simulink library "Tetris_Lib"  (R2023a)
settings: Solver=ode45  StartTime=0.0  StopTime=10.0  RelTol=1e-3  EnableMultiTasking=on
libraries: simulink_extras x33, $bdroot x16, Bit_Multiplexers_Lib x9, Decoders_Lib x4
(part 2 of 2)

== system Tetris_Lib/Trash_Bin/Shape_Bitmaps/L1-shape (180deg) ==
  note: X
      |
      | Y
      |
      | 0
      | 1
      | 2
      | 3
      |
      | 0
      |
      | 1
      |
      | 2
      |
      | 3
  x3(1b) : Inport
  x2(1b) : Inport  Port=2
  x1(1b) : Inport  Port=3
  x0(1b) : Inport  Port=4
  y3(1b) : Inport  Port=5
  y2(1b) : Inport  Port=6
  y1(1b) : Inport  Port=7
  y0(1b) : Inport  Port=8
  And{,1..3,5..16} (16 alike) : Logic  Inputs=3  IconShape=distinctive  AllPortsSameDT=off  OutDataTypeStr=boolean
  And4 : Logic  Operator=OR  Inputs=16  IconShape=distinctive  AllPortsSameDT=off  OutDataTypeStr=boolean
  None{1..4,8..9,11..16} (12 alike) : Constant  Value=0  OutDataTypeStr=boolean
  None{5..7,10} (4 alike) : Constant  OutDataTypeStr=boolean
  Out(1b) : Outport
  wires:
  y0(1b)/1 -> And/3, And1/3, And6/3, And5/3
  y1(1b)/1 -> And2/3, And3/3, And8/3, And7/3
  x0(1b)/1 -> And/2, And2/2, And11/2, And9/2
  x1(1b)/1 -> And1/2, And3/2, And12/2, And10/2
  And4/1 -> Out(1b)/1
  x2(1b)/1 -> And5/2, And7/2, And15/2, And13/2
  x3(1b)/1 -> And6/2, And8/2, And16/2, And14/2
  y2(1b)/1 -> And9/3, And10/3, And14/3, And13/3
  y3(1b)/1 -> And11/3, And12/3, And16/3, And15/3
  And6/1 -> And4/1
  And5/1 -> And4/2
  And1/1 -> And4/3
  And/1 -> And4/4
  And8/1 -> And4/5
  And7/1 -> And4/6
  And3/1 -> And4/7
  And2/1 -> And4/8
  And14/1 -> And4/9
  And13/1 -> And4/10
  And10/1 -> And4/11
  And9/1 -> And4/12
  And16/1 -> And4/13
  And15/1 -> And4/14
  And12/1 -> And4/15
  And11/1 -> And4/16
  None10/1 -> And/1
  None1/1 -> And2/1
  None2/1 -> And9/1
  None3/1 -> And11/1
  None4/1 -> And12/1
  None5/1 -> And10/1
  None6/1 -> And3/1
  None7/1 -> And1/1
  None8/1 -> And5/1
  None9/1 -> And7/1
  None11/1 -> And13/1
  None12/1 -> And15/1
  None13/1 -> And6/1
  None14/1 -> And8/1
  None15/1 -> And14/1
  None16/1 -> And16/1

== system Tetris_Lib/Trash_Bin/Shape_Bitmaps/L1-shape (270deg) ==
  note: X
      |
      | Y
      |
      | 0
      | 1
      | 2
      | 3
      |
      | 0
      |
      | 1
      |
      | 2
      |
      | 3
  x3(1b) : Inport
  x2(1b) : Inport  Port=2
  x1(1b) : Inport  Port=3
  x0(1b) : Inport  Port=4
  y3(1b) : Inport  Port=5
  y2(1b) : Inport  Port=6
  y1(1b) : Inport  Port=7
  y0(1b) : Inport  Port=8
  And{,1..3,5..16} (16 alike) : Logic  Inputs=3  IconShape=distinctive  AllPortsSameDT=off  OutDataTypeStr=boolean
  And4 : Logic  Operator=OR  Inputs=16  IconShape=distinctive  AllPortsSameDT=off  OutDataTypeStr=boolean
  None{1,6,8..9} (4 alike) : Constant  OutDataTypeStr=boolean
  None{2..5,7,10..16} (12 alike) : Constant  Value=0  OutDataTypeStr=boolean
  Out(1b) : Outport
  wires:
  y0(1b)/1 -> And/3, And1/3, And6/3, And5/3
  y1(1b)/1 -> And2/3, And3/3, And8/3, And7/3
  x0(1b)/1 -> And/2, And2/2, And11/2, And9/2
  x1(1b)/1 -> And1/2, And3/2, And12/2, And10/2
  And4/1 -> Out(1b)/1
  x2(1b)/1 -> And5/2, And7/2, And15/2, And13/2
  x3(1b)/1 -> And6/2, And8/2, And16/2, And14/2
  y2(1b)/1 -> And9/3, And10/3, And14/3, And13/3
  y3(1b)/1 -> And11/3, And12/3, And16/3, And15/3
  And6/1 -> And4/1
  And5/1 -> And4/2
  And1/1 -> And4/3
  And/1 -> And4/4
  And8/1 -> And4/5
  And7/1 -> And4/6
  And3/1 -> And4/7
  And2/1 -> And4/8
  And14/1 -> And4/9
  And13/1 -> And4/10
  And10/1 -> And4/11
  And9/1 -> And4/12
  And16/1 -> And4/13
  And15/1 -> And4/14
  And12/1 -> And4/15
  And11/1 -> And4/16
  None10/1 -> And/1
  None1/1 -> And2/1
  None2/1 -> And9/1
  None3/1 -> And11/1
  None4/1 -> And12/1
  None5/1 -> And10/1
  None6/1 -> And3/1
  None7/1 -> And1/1
  None8/1 -> And5/1
  None9/1 -> And7/1
  None11/1 -> And13/1
  None12/1 -> And15/1
  None13/1 -> And6/1
  None14/1 -> And8/1
  None15/1 -> And14/1
  None16/1 -> And16/1

== system Tetris_Lib/Trash_Bin/Shape_Bitmaps/L1-shape (90deg) ==
  note: X
      |
      | Y
      |
      | 0
      | 1
      | 2
      | 3
      |
      | 0
      |
      | 1
      |
      | 2
      |
      | 3
  x3(1b) : Inport
  x2(1b) : Inport  Port=2
  x1(1b) : Inport  Port=3
  x0(1b) : Inport  Port=4
  y3(1b) : Inport  Port=5
  y2(1b) : Inport  Port=6
  y1(1b) : Inport  Port=7
  y0(1b) : Inport  Port=8
  And{,1..3,5..16} (16 alike) : Logic  Inputs=3  IconShape=distinctive  AllPortsSameDT=off  OutDataTypeStr=boolean
  And4 : Logic  Operator=OR  Inputs=16  IconShape=distinctive  AllPortsSameDT=off  OutDataTypeStr=boolean
  None{1,7..8,10} (4 alike) : Constant  OutDataTypeStr=boolean
  None{2..6,9,11..16} (12 alike) : Constant  Value=0  OutDataTypeStr=boolean
  Out(1b) : Outport
  wires:
  y0(1b)/1 -> And/3, And1/3, And6/3, And5/3
  y1(1b)/1 -> And2/3, And3/3, And8/3, And7/3
  x0(1b)/1 -> And/2, And2/2, And11/2, And9/2
  x1(1b)/1 -> And1/2, And3/2, And12/2, And10/2
  And4/1 -> Out(1b)/1
  x2(1b)/1 -> And5/2, And7/2, And15/2, And13/2
  x3(1b)/1 -> And6/2, And8/2, And16/2, And14/2
  y2(1b)/1 -> And9/3, And10/3, And14/3, And13/3
  y3(1b)/1 -> And11/3, And12/3, And16/3, And15/3
  And6/1 -> And4/1
  And5/1 -> And4/2
  And1/1 -> And4/3
  And/1 -> And4/4
  And8/1 -> And4/5
  And7/1 -> And4/6
  And3/1 -> And4/7
  And2/1 -> And4/8
  And14/1 -> And4/9
  And13/1 -> And4/10
  And10/1 -> And4/11
  And9/1 -> And4/12
  And16/1 -> And4/13
  And15/1 -> And4/14
  And12/1 -> And4/15
  And11/1 -> And4/16
  None10/1 -> And/1
  None1/1 -> And2/1
  None2/1 -> And9/1
  None3/1 -> And11/1
  None4/1 -> And12/1
  None5/1 -> And10/1
  None6/1 -> And3/1
  None7/1 -> And1/1
  None8/1 -> And5/1
  None9/1 -> And7/1
  None11/1 -> And13/1
  None12/1 -> And15/1
  None13/1 -> And6/1
  None14/1 -> And8/1
  None15/1 -> And14/1
  None16/1 -> And16/1

== system Tetris_Lib/Trash_Bin/Shape_Bitmaps/L2-shape (0deg) ==
  note: X
      |
      | Y
      |
      | 0
      | 1
      | 2
      | 3
      |
      | 0
      |
      | 1
      |
      | 2
      |
      | 3
  x3(1b) : Inport
  x2(1b) : Inport  Port=2
  x1(1b) : Inport  Port=3
  x0(1b) : Inport  Port=4
  y3(1b) : Inport  Port=5
  y2(1b) : Inport  Port=6
  y1(1b) : Inport  Port=7
  y0(1b) : Inport  Port=8
  And{,1..3,5..16} (16 alike) : Logic  Inputs=3  IconShape=distinctive  AllPortsSameDT=off  OutDataTypeStr=boolean
  And4 : Logic  Operator=OR  Inputs=16  IconShape=distinctive  AllPortsSameDT=off  OutDataTypeStr=boolean
  None{1,3..4,8..16} (12 alike) : Constant  Value=0  OutDataTypeStr=boolean
  None{2,5..7} (4 alike) : Constant  OutDataTypeStr=boolean
  Out(1b) : Outport
  wires:
  y0(1b)/1 -> And/3, And1/3, And6/3, And5/3
  y1(1b)/1 -> And2/3, And3/3, And8/3, And7/3
  x0(1b)/1 -> And/2, And2/2, And11/2, And9/2
  x1(1b)/1 -> And1/2, And3/2, And12/2, And10/2
  And4/1 -> Out(1b)/1
  x2(1b)/1 -> And5/2, And7/2, And15/2, And13/2
  x3(1b)/1 -> And6/2, And8/2, And16/2, And14/2
  y2(1b)/1 -> And9/3, And10/3, And14/3, And13/3
  y3(1b)/1 -> And11/3, And12/3, And16/3, And15/3
  And6/1 -> And4/1
  And5/1 -> And4/2
  And1/1 -> And4/3
  And/1 -> And4/4
  And8/1 -> And4/5
  And7/1 -> And4/6
  And3/1 -> And4/7
  And2/1 -> And4/8
  And14/1 -> And4/9
  And13/1 -> And4/10
  And10/1 -> And4/11
  And9/1 -> And4/12
  And16/1 -> And4/13
  And15/1 -> And4/14
  And12/1 -> And4/15
  And11/1 -> And4/16
  None10/1 -> And/1
  None1/1 -> And2/1
  None2/1 -> And9/1
  None3/1 -> And11/1
  None4/1 -> And12/1
  None5/1 -> And10/1
  None6/1 -> And3/1
  None7/1 -> And1/1
  None8/1 -> And5/1
  None9/1 -> And7/1
  None11/1 -> And13/1
  None12/1 -> And15/1
  None13/1 -> And6/1
  None14/1 -> And8/1
  None15/1 -> And14/1
  None16/1 -> And16/1

== system Tetris_Lib/Trash_Bin/Shape_Bitmaps/L2-shape (180deg) ==
  note: X
      |
      | Y
      |
      | 0
      | 1
      | 2
      | 3
      |
      | 0
      |
      | 1
      |
      | 2
      |
      | 3
  x3(1b) : Inport
  x2(1b) : Inport  Port=2
  x1(1b) : Inport  Port=3
  x0(1b) : Inport  Port=4
  y3(1b) : Inport  Port=5
  y2(1b) : Inport  Port=6
  y1(1b) : Inport  Port=7
  y0(1b) : Inport  Port=8
  And{,1..3,5..16} (16 alike) : Logic  Inputs=3  IconShape=distinctive  AllPortsSameDT=off  OutDataTypeStr=boolean
  And4 : Logic  Operator=OR  Inputs=16  IconShape=distinctive  AllPortsSameDT=off  OutDataTypeStr=boolean
  None{1..2,7,10} (4 alike) : Constant  OutDataTypeStr=boolean
  None{3..6,8..9,11..16} (12 alike) : Constant  Value=0  OutDataTypeStr=boolean
  Out(1b) : Outport
  wires:
  y0(1b)/1 -> And/3, And1/3, And6/3, And5/3
  y1(1b)/1 -> And2/3, And3/3, And8/3, And7/3
  x0(1b)/1 -> And/2, And2/2, And11/2, And9/2
  x1(1b)/1 -> And1/2, And3/2, And12/2, And10/2
  And4/1 -> Out(1b)/1
  x2(1b)/1 -> And5/2, And7/2, And15/2, And13/2
  x3(1b)/1 -> And6/2, And8/2, And16/2, And14/2
  y2(1b)/1 -> And9/3, And10/3, And14/3, And13/3
  y3(1b)/1 -> And11/3, And12/3, And16/3, And15/3
  And6/1 -> And4/1
  And5/1 -> And4/2
  And1/1 -> And4/3
  And/1 -> And4/4
  And8/1 -> And4/5
  And7/1 -> And4/6
  And3/1 -> And4/7
  And2/1 -> And4/8
  And14/1 -> And4/9
  And13/1 -> And4/10
  And10/1 -> And4/11
  And9/1 -> And4/12
  And16/1 -> And4/13
  And15/1 -> And4/14
  And12/1 -> And4/15
  And11/1 -> And4/16
  None10/1 -> And/1
  None1/1 -> And2/1
  None2/1 -> And9/1
  None3/1 -> And11/1
  None4/1 -> And12/1
  None5/1 -> And10/1
  None6/1 -> And3/1
  None7/1 -> And1/1
  None8/1 -> And5/1
  None9/1 -> And7/1
  None11/1 -> And13/1
  None12/1 -> And15/1
  None13/1 -> And6/1
  None14/1 -> And8/1
  None15/1 -> And14/1
  None16/1 -> And16/1

== system Tetris_Lib/Trash_Bin/Shape_Bitmaps/L2-shape (270deg) ==
  note: X
      |
      | Y
      |
      | 0
      | 1
      | 2
      | 3
      |
      | 0
      |
      | 1
      |
      | 2
      |
      | 3
  x3(1b) : Inport
  x2(1b) : Inport  Port=2
  x1(1b) : Inport  Port=3
  x0(1b) : Inport  Port=4
  y3(1b) : Inport  Port=5
  y2(1b) : Inport  Port=6
  y1(1b) : Inport  Port=7
  y0(1b) : Inport  Port=8
  And{,1..3,5..16} (16 alike) : Logic  Inputs=3  IconShape=distinctive  AllPortsSameDT=off  OutDataTypeStr=boolean
  And4 : Logic  Operator=OR  Inputs=16  IconShape=distinctive  AllPortsSameDT=off  OutDataTypeStr=boolean
  None{1..6,11..16} (12 alike) : Constant  Value=0  OutDataTypeStr=boolean
  None{7..10} (4 alike) : Constant  OutDataTypeStr=boolean
  Out(1b) : Outport
  wires:
  y0(1b)/1 -> And/3, And1/3, And6/3, And5/3
  y1(1b)/1 -> And2/3, And3/3, And8/3, And7/3
  x0(1b)/1 -> And/2, And2/2, And11/2, And9/2
  x1(1b)/1 -> And1/2, And3/2, And12/2, And10/2
  And4/1 -> Out(1b)/1
  x2(1b)/1 -> And5/2, And7/2, And15/2, And13/2
  x3(1b)/1 -> And6/2, And8/2, And16/2, And14/2
  y2(1b)/1 -> And9/3, And10/3, And14/3, And13/3
  y3(1b)/1 -> And11/3, And12/3, And16/3, And15/3
  And6/1 -> And4/1
  And5/1 -> And4/2
  And1/1 -> And4/3
  And/1 -> And4/4
  And8/1 -> And4/5
  And7/1 -> And4/6
  And3/1 -> And4/7
  And2/1 -> And4/8
  And14/1 -> And4/9
  And13/1 -> And4/10
  And10/1 -> And4/11
  And9/1 -> And4/12
  And16/1 -> And4/13
  And15/1 -> And4/14
  And12/1 -> And4/15
  And11/1 -> And4/16
  None10/1 -> And/1
  None1/1 -> And2/1
  None2/1 -> And9/1
  None3/1 -> And11/1
  None4/1 -> And12/1
  None5/1 -> And10/1
  None6/1 -> And3/1
  None7/1 -> And1/1
  None8/1 -> And5/1
  None9/1 -> And7/1
  None11/1 -> And13/1
  None12/1 -> And15/1
  None13/1 -> And6/1
  None14/1 -> And8/1
  None15/1 -> And14/1
  None16/1 -> And16/1

== system Tetris_Lib/Trash_Bin/Shape_Bitmaps/L2-shape (90deg) ==
  note: X
      |
      | Y
      |
      | 0
      | 1
      | 2
      | 3
      |
      | 0
      |
      | 1
      |
      | 2
      |
      | 3
  x3(1b) : Inport
  x2(1b) : Inport  Port=2
  x1(1b) : Inport  Port=3
  x0(1b) : Inport  Port=4
  y3(1b) : Inport  Port=5
  y2(1b) : Inport  Port=6
  y1(1b) : Inport  Port=7
  y0(1b) : Inport  Port=8
  And{,1..3,5..16} (16 alike) : Logic  Inputs=3  IconShape=distinctive  AllPortsSameDT=off  OutDataTypeStr=boolean
  And4 : Logic  Operator=OR  Inputs=16  IconShape=distinctive  AllPortsSameDT=off  OutDataTypeStr=boolean
  None{1,6,9..10} (4 alike) : Constant  OutDataTypeStr=boolean
  None{2..5,7..8,11..16} (12 alike) : Constant  Value=0  OutDataTypeStr=boolean
  Out(1b) : Outport
  wires:
  y0(1b)/1 -> And/3, And1/3, And6/3, And5/3
  y1(1b)/1 -> And2/3, And3/3, And8/3, And7/3
  x0(1b)/1 -> And/2, And2/2, And11/2, And9/2
  x1(1b)/1 -> And1/2, And3/2, And12/2, And10/2
  And4/1 -> Out(1b)/1
  x2(1b)/1 -> And5/2, And7/2, And15/2, And13/2
  x3(1b)/1 -> And6/2, And8/2, And16/2, And14/2
  y2(1b)/1 -> And9/3, And10/3, And14/3, And13/3
  y3(1b)/1 -> And11/3, And12/3, And16/3, And15/3
  And6/1 -> And4/1
  And5/1 -> And4/2
  And1/1 -> And4/3
  And/1 -> And4/4
  And8/1 -> And4/5
  And7/1 -> And4/6
  And3/1 -> And4/7
  And2/1 -> And4/8
  And14/1 -> And4/9
  And13/1 -> And4/10
  And10/1 -> And4/11
  And9/1 -> And4/12
  And16/1 -> And4/13
  And15/1 -> And4/14
  And12/1 -> And4/15
  And11/1 -> And4/16
  None10/1 -> And/1
  None1/1 -> And2/1
  None2/1 -> And9/1
  None3/1 -> And11/1
  None4/1 -> And12/1
  None5/1 -> And10/1
  None6/1 -> And3/1
  None7/1 -> And1/1
  None8/1 -> And5/1
  None9/1 -> And7/1
  None11/1 -> And13/1
  None12/1 -> And15/1
  None13/1 -> And6/1
  None14/1 -> And8/1
  None15/1 -> And14/1
  None16/1 -> And16/1

== system Tetris_Lib/Trash_Bin/Shape_Bitmaps/O-shape ==
  note: X
      |
      | Y
      |
      | 0
      | 1
      | 2
      | 3
      |
      | 0
      |
      | 1
      |
      | 2
      |
      | 3
  x3(1b) : Inport
  x2(1b) : Inport  Port=2
  x1(1b) : Inport  Port=3
  x0(1b) : Inport  Port=4
  y3(1b) : Inport  Port=5
  y2(1b) : Inport  Port=6
  y1(1b) : Inport  Port=7
  y0(1b) : Inport  Port=8
  And{,1..3,5..16} (16 alike) : Logic  Inputs=3  IconShape=distinctive  AllPortsSameDT=off  OutDataTypeStr=boolean
  And4 : Logic  Operator=OR  Inputs=16  IconShape=distinctive  AllPortsSameDT=off  OutDataTypeStr=boolean
  None{1,6..7,10} (4 alike) : Constant  OutDataTypeStr=boolean
  None{2..5,8..9,11..16} (12 alike) : Constant  Value=0  OutDataTypeStr=boolean
  Out(1b) : Outport
  wires:
  y0(1b)/1 -> And/3, And1/3, And6/3, And5/3
  y1(1b)/1 -> And2/3, And3/3, And8/3, And7/3
  x0(1b)/1 -> And/2, And2/2, And11/2, And9/2
  x1(1b)/1 -> And1/2, And3/2, And12/2, And10/2
  And4/1 -> Out(1b)/1
  x2(1b)/1 -> And5/2, And7/2, And15/2, And13/2
  x3(1b)/1 -> And6/2, And8/2, And16/2, And14/2
  y2(1b)/1 -> And9/3, And10/3, And14/3, And13/3
  y3(1b)/1 -> And11/3, And12/3, And16/3, And15/3
  And6/1 -> And4/1
  And5/1 -> And4/2
  And1/1 -> And4/3
  And/1 -> And4/4
  And8/1 -> And4/5
  And7/1 -> And4/6
  And3/1 -> And4/7
  And2/1 -> And4/8
  And14/1 -> And4/9
  And13/1 -> And4/10
  And10/1 -> And4/11
  And9/1 -> And4/12
  And16/1 -> And4/13
  And15/1 -> And4/14
  And12/1 -> And4/15
  And11/1 -> And4/16
  None10/1 -> And/1
  None1/1 -> And2/1
  None2/1 -> And9/1
  None3/1 -> And11/1
  None4/1 -> And12/1
  None5/1 -> And10/1
  None6/1 -> And3/1
  None7/1 -> And1/1
  None8/1 -> And5/1
  None9/1 -> And7/1
  None11/1 -> And13/1
  None12/1 -> And15/1
  None13/1 -> And6/1
  None14/1 -> And8/1
  None15/1 -> And14/1
  None16/1 -> And16/1

== system Tetris_Lib/Trash_Bin/Shape_Bitmaps/T-shape (0deg) ==
  note: X
      |
      | Y
      |
      | 0
      | 1
      | 2
      | 3
      |
      | 0
      |
      | 1
      |
      | 2
      |
      | 3
  x3(1b) : Inport
  x2(1b) : Inport  Port=2
  x1(1b) : Inport  Port=3
  x0(1b) : Inport  Port=4
  y3(1b) : Inport  Port=5
  y2(1b) : Inport  Port=6
  y1(1b) : Inport  Port=7
  y0(1b) : Inport  Port=8
  And{,1..3,5..16} (16 alike) : Logic  Inputs=3  IconShape=distinctive  AllPortsSameDT=off  OutDataTypeStr=boolean
  And4 : Logic  Operator=OR  Inputs=16  IconShape=distinctive  AllPortsSameDT=off  OutDataTypeStr=boolean
  None{1..5,9,11..16} (12 alike) : Constant  Value=0  OutDataTypeStr=boolean
  None{6..8,10} (4 alike) : Constant  OutDataTypeStr=boolean
  Out(1b) : Outport
  wires:
  y0(1b)/1 -> And/3, And1/3, And6/3, And5/3
  y1(1b)/1 -> And2/3, And3/3, And8/3, And7/3
  x0(1b)/1 -> And/2, And2/2, And11/2, And9/2
  x1(1b)/1 -> And1/2, And3/2, And12/2, And10/2
  And4/1 -> Out(1b)/1
  x2(1b)/1 -> And5/2, And7/2, And15/2, And13/2
  x3(1b)/1 -> And6/2, And8/2, And16/2, And14/2
  y2(1b)/1 -> And9/3, And10/3, And14/3, And13/3
  y3(1b)/1 -> And11/3, And12/3, And16/3, And15/3
  And6/1 -> And4/1
  And5/1 -> And4/2
  And1/1 -> And4/3
  And/1 -> And4/4
  And8/1 -> And4/5
  And7/1 -> And4/6
  And3/1 -> And4/7
  And2/1 -> And4/8
  And14/1 -> And4/9
  And13/1 -> And4/10
  And10/1 -> And4/11
  And9/1 -> And4/12
  And16/1 -> And4/13
  And15/1 -> And4/14
  And12/1 -> And4/15
  And11/1 -> And4/16
  None10/1 -> And/1
  None1/1 -> And2/1
  None2/1 -> And9/1
  None3/1 -> And11/1
  None4/1 -> And12/1
  None5/1 -> And10/1
  None6/1 -> And3/1
  None7/1 -> And1/1
  None8/1 -> And5/1
  None9/1 -> And7/1
  None11/1 -> And13/1
  None12/1 -> And15/1
  None13/1 -> And6/1
  None14/1 -> And8/1
  None15/1 -> And14/1
  None16/1 -> And16/1

== system Tetris_Lib/Trash_Bin/Shape_Bitmaps/T-shape (180deg) ==
  note: X
      |
      | Y
      |
      | 0
      | 1
      | 2
      | 3
      |
      | 0
      |
      | 1
      |
      | 2
      |
      | 3
  x3(1b) : Inport
  x2(1b) : Inport  Port=2
  x1(1b) : Inport  Port=3
  x0(1b) : Inport  Port=4
  y3(1b) : Inport  Port=5
  y2(1b) : Inport  Port=6
  y1(1b) : Inport  Port=7
  y0(1b) : Inport  Port=8
  And{,1..3,5..16} (16 alike) : Logic  Inputs=3  IconShape=distinctive  AllPortsSameDT=off  OutDataTypeStr=boolean
  And4 : Logic  Operator=OR  Inputs=16  IconShape=distinctive  AllPortsSameDT=off  OutDataTypeStr=boolean
  None{1,6..7,9} (4 alike) : Constant  OutDataTypeStr=boolean
  None{2..5,8,10..16} (12 alike) : Constant  Value=0  OutDataTypeStr=boolean
  Out(1b) : Outport
  wires:
  y0(1b)/1 -> And/3, And1/3, And6/3, And5/3
  y1(1b)/1 -> And2/3, And3/3, And8/3, And7/3
  x0(1b)/1 -> And/2, And2/2, And11/2, And9/2
  x1(1b)/1 -> And1/2, And3/2, And12/2, And10/2
  And4/1 -> Out(1b)/1
  x2(1b)/1 -> And5/2, And7/2, And15/2, And13/2
  x3(1b)/1 -> And6/2, And8/2, And16/2, And14/2
  y2(1b)/1 -> And9/3, And10/3, And14/3, And13/3
  y3(1b)/1 -> And11/3, And12/3, And16/3, And15/3
  And6/1 -> And4/1
  And5/1 -> And4/2
  And1/1 -> And4/3
  And/1 -> And4/4
  And8/1 -> And4/5
  And7/1 -> And4/6
  And3/1 -> And4/7
  And2/1 -> And4/8
  And14/1 -> And4/9
  And13/1 -> And4/10
  And10/1 -> And4/11
  And9/1 -> And4/12
  And16/1 -> And4/13
  And15/1 -> And4/14
  And12/1 -> And4/15
  And11/1 -> And4/16
  None10/1 -> And/1
  None1/1 -> And2/1
  None2/1 -> And9/1
  None3/1 -> And11/1
  None4/1 -> And12/1
  None5/1 -> And10/1
  None6/1 -> And3/1
  None7/1 -> And1/1
  None8/1 -> And5/1
  None9/1 -> And7/1
  None11/1 -> And13/1
  None12/1 -> And15/1
  None13/1 -> And6/1
  None14/1 -> And8/1
  None15/1 -> And14/1
  None16/1 -> And16/1

== system Tetris_Lib/Trash_Bin/Shape_Bitmaps/T-shape (270deg) ==
  note: X
      |
      | Y
      |
      | 0
      | 1
      | 2
      | 3
      |
      | 0
      |
      | 1
      |
      | 2
      |
      | 3
  x3(1b) : Inport
  x2(1b) : Inport  Port=2
  x1(1b) : Inport  Port=3
  x0(1b) : Inport  Port=4
  y3(1b) : Inport  Port=5
  y2(1b) : Inport  Port=6
  y1(1b) : Inport  Port=7
  y0(1b) : Inport  Port=8
  And{,1..3,5..16} (16 alike) : Logic  Inputs=3  IconShape=distinctive  AllPortsSameDT=off  OutDataTypeStr=boolean
  And4 : Logic  Operator=OR  Inputs=16  IconShape=distinctive  AllPortsSameDT=off  OutDataTypeStr=boolean
  None{1..2,6,10} (4 alike) : Constant  OutDataTypeStr=boolean
  None{3..5,7..9,11..16} (12 alike) : Constant  Value=0  OutDataTypeStr=boolean
  Out(1b) : Outport
  wires:
  y0(1b)/1 -> And/3, And1/3, And6/3, And5/3
  y1(1b)/1 -> And2/3, And3/3, And8/3, And7/3
  x0(1b)/1 -> And/2, And2/2, And11/2, And9/2
  x1(1b)/1 -> And1/2, And3/2, And12/2, And10/2
  And4/1 -> Out(1b)/1
  x2(1b)/1 -> And5/2, And7/2, And15/2, And13/2
  x3(1b)/1 -> And6/2, And8/2, And16/2, And14/2
  y2(1b)/1 -> And9/3, And10/3, And14/3, And13/3
  y3(1b)/1 -> And11/3, And12/3, And16/3, And15/3
  And6/1 -> And4/1
  And5/1 -> And4/2
  And1/1 -> And4/3
  And/1 -> And4/4
  And8/1 -> And4/5
  And7/1 -> And4/6
  And3/1 -> And4/7
  And2/1 -> And4/8
  And14/1 -> And4/9
  And13/1 -> And4/10
  And10/1 -> And4/11
  And9/1 -> And4/12
  And16/1 -> And4/13
  And15/1 -> And4/14
  And12/1 -> And4/15
  And11/1 -> And4/16
  None10/1 -> And/1
  None1/1 -> And2/1
  None2/1 -> And9/1
  None3/1 -> And11/1
  None4/1 -> And12/1
  None5/1 -> And10/1
  None6/1 -> And3/1
  None7/1 -> And1/1
  None8/1 -> And5/1
  None9/1 -> And7/1
  None11/1 -> And13/1
  None12/1 -> And15/1
  None13/1 -> And6/1
  None14/1 -> And8/1
  None15/1 -> And14/1
  None16/1 -> And16/1

== system Tetris_Lib/Trash_Bin/Shape_Bitmaps/T-shape (90deg) ==
  note: X
      |
      | Y
      |
      | 0
      | 1
      | 2
      | 3
      |
      | 0
      |
      | 1
      |
      | 2
      |
      | 3
  x3(1b) : Inport
  x2(1b) : Inport  Port=2
  x1(1b) : Inport  Port=3
  x0(1b) : Inport  Port=4
  y3(1b) : Inport  Port=5
  y2(1b) : Inport  Port=6
  y1(1b) : Inport  Port=7
  y0(1b) : Inport  Port=8
  And{,1..3,5..16} (16 alike) : Logic  Inputs=3  IconShape=distinctive  AllPortsSameDT=off  OutDataTypeStr=boolean
  And4 : Logic  Operator=OR  Inputs=16  IconShape=distinctive  AllPortsSameDT=off  OutDataTypeStr=boolean
  None{1,5..7} (4 alike) : Constant  OutDataTypeStr=boolean
  None{2..4,8..16} (12 alike) : Constant  Value=0  OutDataTypeStr=boolean
  Out(1b) : Outport
  wires:
  y0(1b)/1 -> And/3, And1/3, And6/3, And5/3
  y1(1b)/1 -> And2/3, And3/3, And8/3, And7/3
  x0(1b)/1 -> And/2, And2/2, And11/2, And9/2
  x1(1b)/1 -> And1/2, And3/2, And12/2, And10/2
  And4/1 -> Out(1b)/1
  x2(1b)/1 -> And5/2, And7/2, And15/2, And13/2
  x3(1b)/1 -> And6/2, And8/2, And16/2, And14/2
  y2(1b)/1 -> And9/3, And10/3, And14/3, And13/3
  y3(1b)/1 -> And11/3, And12/3, And16/3, And15/3
  And6/1 -> And4/1
  And5/1 -> And4/2
  And1/1 -> And4/3
  And/1 -> And4/4
  And8/1 -> And4/5
  And7/1 -> And4/6
  And3/1 -> And4/7
  And2/1 -> And4/8
  And14/1 -> And4/9
  And13/1 -> And4/10
  And10/1 -> And4/11
  And9/1 -> And4/12
  And16/1 -> And4/13
  And15/1 -> And4/14
  And12/1 -> And4/15
  And11/1 -> And4/16
  None10/1 -> And/1
  None1/1 -> And2/1
  None2/1 -> And9/1
  None3/1 -> And11/1
  None4/1 -> And12/1
  None5/1 -> And10/1
  None6/1 -> And3/1
  None7/1 -> And1/1
  None8/1 -> And5/1
  None9/1 -> And7/1
  None11/1 -> And13/1
  None12/1 -> And15/1
  None13/1 -> And6/1
  None14/1 -> And8/1
  None15/1 -> And14/1
  None16/1 -> And16/1

== system Tetris_Lib/Trash_Bin/Shape_Bitmaps/Z1-shape (0deg) ==
  note: X
      |
      | Y
      |
      | 0
      | 1
      | 2
      | 3
      |
      | 0
      |
      | 1
      |
      | 2
      |
      | 3
  x3(1b) : Inport
  x2(1b) : Inport  Port=2
  x1(1b) : Inport  Port=3
  x0(1b) : Inport  Port=4
  y3(1b) : Inport  Port=5
  y2(1b) : Inport  Port=6
  y1(1b) : Inport  Port=7
  y0(1b) : Inport  Port=8
  And{,1..3,5..16} (16 alike) : Logic  Inputs=3  IconShape=distinctive  AllPortsSameDT=off  OutDataTypeStr=boolean
  And4 : Logic  Operator=OR  Inputs=16  IconShape=distinctive  AllPortsSameDT=off  OutDataTypeStr=boolean
  None{1..5,8,11..16} (12 alike) : Constant  Value=0  OutDataTypeStr=boolean
  None{6..7,9..10} (4 alike) : Constant  OutDataTypeStr=boolean
  Out(1b) : Outport
  wires:
  y0(1b)/1 -> And/3, And1/3, And6/3, And5/3
  y1(1b)/1 -> And2/3, And3/3, And8/3, And7/3
  x0(1b)/1 -> And/2, And2/2, And11/2, And9/2
  x1(1b)/1 -> And1/2, And3/2, And12/2, And10/2
  And4/1 -> Out(1b)/1
  x2(1b)/1 -> And5/2, And7/2, And15/2, And13/2
  x3(1b)/1 -> And6/2, And8/2, And16/2, And14/2
  y2(1b)/1 -> And9/3, And10/3, And14/3, And13/3
  y3(1b)/1 -> And11/3, And12/3, And16/3, And15/3
  And6/1 -> And4/1
  And5/1 -> And4/2
  And1/1 -> And4/3
  And/1 -> And4/4
  And8/1 -> And4/5
  And7/1 -> And4/6
  And3/1 -> And4/7
  And2/1 -> And4/8
  And14/1 -> And4/9
  And13/1 -> And4/10
  And10/1 -> And4/11
  And9/1 -> And4/12
  And16/1 -> And4/13
  And15/1 -> And4/14
  And12/1 -> And4/15
  And11/1 -> And4/16
  None10/1 -> And/1
  None1/1 -> And2/1
  None2/1 -> And9/1
  None3/1 -> And11/1
  None4/1 -> And12/1
  None5/1 -> And10/1
  None6/1 -> And3/1
  None7/1 -> And1/1
  None8/1 -> And5/1
  None9/1 -> And7/1
  None11/1 -> And13/1
  None12/1 -> And15/1
  None13/1 -> And6/1
  None14/1 -> And8/1
  None15/1 -> And14/1
  None16/1 -> And16/1

== system Tetris_Lib/Trash_Bin/Shape_Bitmaps/Z1-shape (90deg) ==
  note: X
      |
      | Y
      |
      | 0
      | 1
      | 2
      | 3
      |
      | 0
      |
      | 1
      |
      | 2
      |
      | 3
  x3(1b) : Inport
  x2(1b) : Inport  Port=2
  x1(1b) : Inport  Port=3
  x0(1b) : Inport  Port=4
  y3(1b) : Inport  Port=5
  y2(1b) : Inport  Port=6
  y1(1b) : Inport  Port=7
  y0(1b) : Inport  Port=8
  And{,1..3,5..16} (16 alike) : Logic  Inputs=3  IconShape=distinctive  AllPortsSameDT=off  OutDataTypeStr=boolean
  And4 : Logic  Operator=OR  Inputs=16  IconShape=distinctive  AllPortsSameDT=off  OutDataTypeStr=boolean
  None{1..2,6..7} (4 alike) : Constant  OutDataTypeStr=boolean
  None{3..5,8..16} (12 alike) : Constant  Value=0  OutDataTypeStr=boolean
  Out(1b) : Outport
  wires:
  y0(1b)/1 -> And/3, And1/3, And6/3, And5/3
  y1(1b)/1 -> And2/3, And3/3, And8/3, And7/3
  x0(1b)/1 -> And/2, And2/2, And11/2, And9/2
  x1(1b)/1 -> And1/2, And3/2, And12/2, And10/2
  And4/1 -> Out(1b)/1
  x2(1b)/1 -> And5/2, And7/2, And15/2, And13/2
  x3(1b)/1 -> And6/2, And8/2, And16/2, And14/2
  y2(1b)/1 -> And9/3, And10/3, And14/3, And13/3
  y3(1b)/1 -> And11/3, And12/3, And16/3, And15/3
  And6/1 -> And4/1
  And5/1 -> And4/2
  And1/1 -> And4/3
  And/1 -> And4/4
  And8/1 -> And4/5
  And7/1 -> And4/6
  And3/1 -> And4/7
  And2/1 -> And4/8
  And14/1 -> And4/9
  And13/1 -> And4/10
  And10/1 -> And4/11
  And9/1 -> And4/12
  And16/1 -> And4/13
  And15/1 -> And4/14
  And12/1 -> And4/15
  And11/1 -> And4/16
  None10/1 -> And/1
  None1/1 -> And2/1
  None2/1 -> And9/1
  None3/1 -> And11/1
  None4/1 -> And12/1
  None5/1 -> And10/1
  None6/1 -> And3/1
  None7/1 -> And1/1
  None8/1 -> And5/1
  None9/1 -> And7/1
  None11/1 -> And13/1
  None12/1 -> And15/1
  None13/1 -> And6/1
  None14/1 -> And8/1
  None15/1 -> And14/1
  None16/1 -> And16/1

== system Tetris_Lib/Trash_Bin/Shape_Bitmaps/Z2-shape (0deg) ==
  note: X
      |
      | Y
      |
      | 0
      | 1
      | 2
      | 3
      |
      | 0
      |
      | 1
      |
      | 2
      |
      | 3
  x3(1b) : Inport
  x2(1b) : Inport  Port=2
  x1(1b) : Inport  Port=3
  x0(1b) : Inport  Port=4
  y3(1b) : Inport  Port=5
  y2(1b) : Inport  Port=6
  y1(1b) : Inport  Port=7
  y0(1b) : Inport  Port=8
  And{,1..3,5..16} (16 alike) : Logic  Inputs=3  IconShape=distinctive  AllPortsSameDT=off  OutDataTypeStr=boolean
  And4 : Logic  Operator=OR  Inputs=16  IconShape=distinctive  AllPortsSameDT=off  OutDataTypeStr=boolean
  None{1,6..8} (4 alike) : Constant  OutDataTypeStr=boolean
  None{2..5,9..16} (12 alike) : Constant  Value=0  OutDataTypeStr=boolean
  Out(1b) : Outport
  wires:
  y0(1b)/1 -> And/3, And1/3, And6/3, And5/3
  y1(1b)/1 -> And2/3, And3/3, And8/3, And7/3
  x0(1b)/1 -> And/2, And2/2, And11/2, And9/2
  x1(1b)/1 -> And1/2, And3/2, And12/2, And10/2
  And4/1 -> Out(1b)/1
  x2(1b)/1 -> And5/2, And7/2, And15/2, And13/2
  x3(1b)/1 -> And6/2, And8/2, And16/2, And14/2
  y2(1b)/1 -> And9/3, And10/3, And14/3, And13/3
  y3(1b)/1 -> And11/3, And12/3, And16/3, And15/3
  And6/1 -> And4/1
  And5/1 -> And4/2
  And1/1 -> And4/3
  And/1 -> And4/4
  And8/1 -> And4/5
  And7/1 -> And4/6
  And3/1 -> And4/7
  And2/1 -> And4/8
  And14/1 -> And4/9
  And13/1 -> And4/10
  And10/1 -> And4/11
  And9/1 -> And4/12
  And16/1 -> And4/13
  And15/1 -> And4/14
  And12/1 -> And4/15
  And11/1 -> And4/16
  None10/1 -> And/1
  None1/1 -> And2/1
  None2/1 -> And9/1
  None3/1 -> And11/1
  None4/1 -> And12/1
  None5/1 -> And10/1
  None6/1 -> And3/1
  None7/1 -> And1/1
  None8/1 -> And5/1
  None9/1 -> And7/1
  None11/1 -> And13/1
  None12/1 -> And15/1
  None13/1 -> And6/1
  None14/1 -> And8/1
  None15/1 -> And14/1
  None16/1 -> And16/1

== system Tetris_Lib/Trash_Bin/Shape_Bitmaps/Z2-shape (90deg) ==
  note: X
      |
      | Y
      |
      | 0
      | 1
      | 2
      | 3
      |
      | 0
      |
      | 1
      |
      | 2
      |
      | 3
  x3(1b) : Inport
  x2(1b) : Inport  Port=2
  x1(1b) : Inport  Port=3
  x0(1b) : Inport  Port=4
  y3(1b) : Inport  Port=5
  y2(1b) : Inport  Port=6
  y1(1b) : Inport  Port=7
  y0(1b) : Inport  Port=8
  And{,1..3,5..16} (16 alike) : Logic  Inputs=3  IconShape=distinctive  AllPortsSameDT=off  OutDataTypeStr=boolean
  And4 : Logic  Operator=OR  Inputs=16  IconShape=distinctive  AllPortsSameDT=off  OutDataTypeStr=boolean
  None{1,5..6,10} (4 alike) : Constant  OutDataTypeStr=boolean
  None{2..4,7..9,11..16} (12 alike) : Constant  Value=0  OutDataTypeStr=boolean
  Out(1b) : Outport
  wires:
  y0(1b)/1 -> And/3, And1/3, And6/3, And5/3
  y1(1b)/1 -> And2/3, And3/3, And8/3, And7/3
  x0(1b)/1 -> And/2, And2/2, And11/2, And9/2
  x1(1b)/1 -> And1/2, And3/2, And12/2, And10/2
  And4/1 -> Out(1b)/1
  x2(1b)/1 -> And5/2, And7/2, And15/2, And13/2
  x3(1b)/1 -> And6/2, And8/2, And16/2, And14/2
  y2(1b)/1 -> And9/3, And10/3, And14/3, And13/3
  y3(1b)/1 -> And11/3, And12/3, And16/3, And15/3
  And6/1 -> And4/1
  And5/1 -> And4/2
  And1/1 -> And4/3
  And/1 -> And4/4
  And8/1 -> And4/5
  And7/1 -> And4/6
  And3/1 -> And4/7
  And2/1 -> And4/8
  And14/1 -> And4/9
  And13/1 -> And4/10
  And10/1 -> And4/11
  And9/1 -> And4/12
  And16/1 -> And4/13
  And15/1 -> And4/14
  And12/1 -> And4/15
  And11/1 -> And4/16
  None10/1 -> And/1
  None1/1 -> And2/1
  None2/1 -> And9/1
  None3/1 -> And11/1
  None4/1 -> And12/1
  None5/1 -> And10/1
  None6/1 -> And3/1
  None7/1 -> And1/1
  None8/1 -> And5/1
  None9/1 -> And7/1
  None11/1 -> And13/1
  None12/1 -> And15/1
  None13/1 -> And6/1
  None14/1 -> And8/1
  None15/1 -> And14/1
  None16/1 -> And16/1
